simulink model "BLOC_ICE_control"  (R2016a)
settings: Solver=VariableStepAuto  StartTime=0.0  StopTime=10.0  RelTol=1e-3
undefined symbols (not defined in the file): DiscIntNeverNeededParam, fa_delta_derating, fa_high_derating_point, fa_kp_idle_tr_off, fa_kp_idle_tr_on, fa_low_derating_point, fa_max_tq_ice, fa_n_ice, fa_taui_idle_tr_off, fa_taui_idle_tr_on, fa_tq_loss, fa_tq_max_speed, hev_dt
libraries: simulink x3
settings Model: Creator=Florent  LastModifiedBy=Florent
settings OptimizationCC: DefaultParameterBehavior=Inlined  OptimizeModelRefInitCode=on  LifeSpan=1
settings RTWCC: SystemTargetFile=ert.tlc  TemplateMakefile=ert_default_tmf  GenerateReport=on  IncludeHyperlinkInReport=on  LaunchReport=on  TargetLang=C++  GenerateTraceInfo=on  GenerateTraceReport=on  GenerateTraceReportSl=on  GenerateTraceReportSf=on  GenerateTraceReportEml=on
settings CodeAppCC: ForceParamTrailComments=on  OperatorAnnotations=on  SimulinkDataObjDesc=on  SFDataObjDesc=on  MATLABFcnDesc=on  InsertBlockDesc=on  MATLABSourceComments=on
settings ERTTargetCC: GenerateSampleERTMain=on  MultiInstanceERTCode=on  CodeInterfacePackaging=C++ class  InlinedParameterPlacement=NonHierarchical  RootIOFormat=Structure reference  ERTCustomFileTemplate=example_file_process.tlc

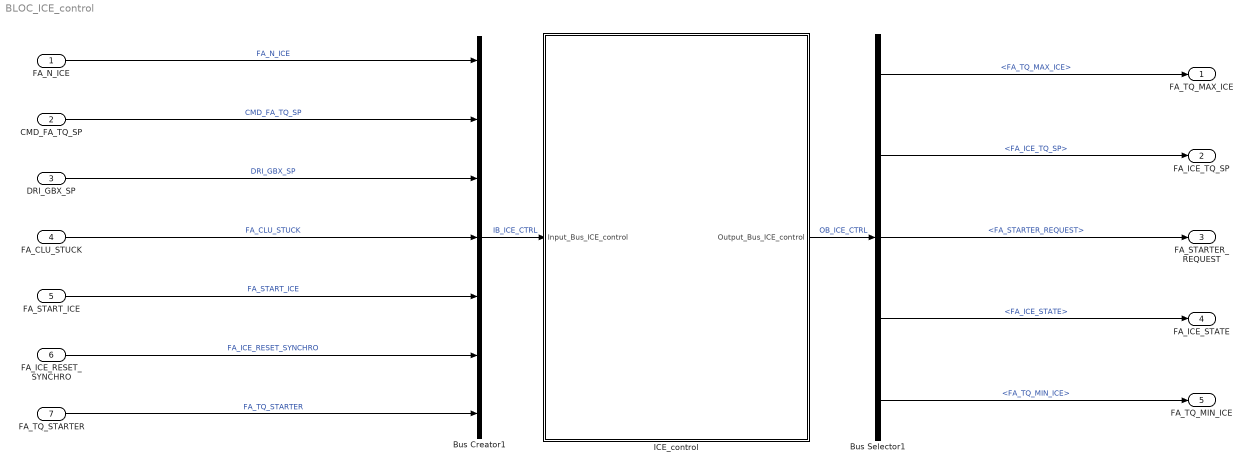
== system BLOC_ICE_control ==
  FA_N_ICE : Inport
  CMD_FA_TQ_SP : Inport  Port=2
  DRI_GBX_SP : Inport  Port=3
  FA_CLU_STUCK : Inport  Port=4
  FA_START_ICE : Inport  Port=5
  FA_ICE_RESET_SYNCHRO : Inport  Port=6
  FA_TQ_STARTER : Inport  Port=7
  Bus Creator1 : BusCreator  Inputs=7
  Bus Selector1 : BusSelector  OutputSignals=FA_TQ_MAX_ICE,FA_ICE_TQ_SP,FA_STARTER_REQUEST,FA_ICE_STATE,FA_TQ_MIN_ICE
  ICE_control : Subsystem  TreatAsAtomicUnit=on  SystemSampleTime=hev_dt
  FA_TQ_MAX_ICE : Outport
  FA_ICE_TQ_SP : Outport  Port=2
  FA_STARTER_REQUEST : Outport  Port=3
  FA_ICE_STATE : Outport  Port=4
  FA_TQ_MIN_ICE : Outport  Port=5
  wires:
  FA_N_ICE/1 -> Bus Creator1/1  "FA_N_ICE"
  CMD_FA_TQ_SP/1 -> Bus Creator1/2  "CMD_FA_TQ_SP"
  DRI_GBX_SP/1 -> Bus Creator1/3  "DRI_GBX_SP"
  FA_CLU_STUCK/1 -> Bus Creator1/4  "FA_CLU_STUCK"
  FA_START_ICE/1 -> Bus Creator1/5  "FA_START_ICE"
  FA_ICE_RESET_SYNCHRO/1 -> Bus Creator1/6  "FA_ICE_RESET_SYNCHRO"
  Bus Creator1/1 -> ICE_control/1("Input_Bus_ICE_control ")  "IB_ICE_CTRL"
  ICE_control/1(Output_Bus_ICE_control) -> Bus Selector1/1  "OB_ICE_CTRL"
  Bus Selector1/1 -> FA_TQ_MAX_ICE/1  "<FA_TQ_MAX_ICE>"
  Bus Selector1/2 -> FA_ICE_TQ_SP/1  "<FA_ICE_TQ_SP>"
  Bus Selector1/3 -> FA_STARTER_REQUEST/1  "<FA_STARTER_REQUEST>"
  Bus Selector1/4 -> FA_ICE_STATE/1  "<FA_ICE_STATE>"
  Bus Selector1/5 -> FA_TQ_MIN_ICE/1  "<FA_TQ_MIN_ICE>"
  FA_TQ_STARTER/1 -> Bus Creator1/7  "FA_TQ_STARTER"

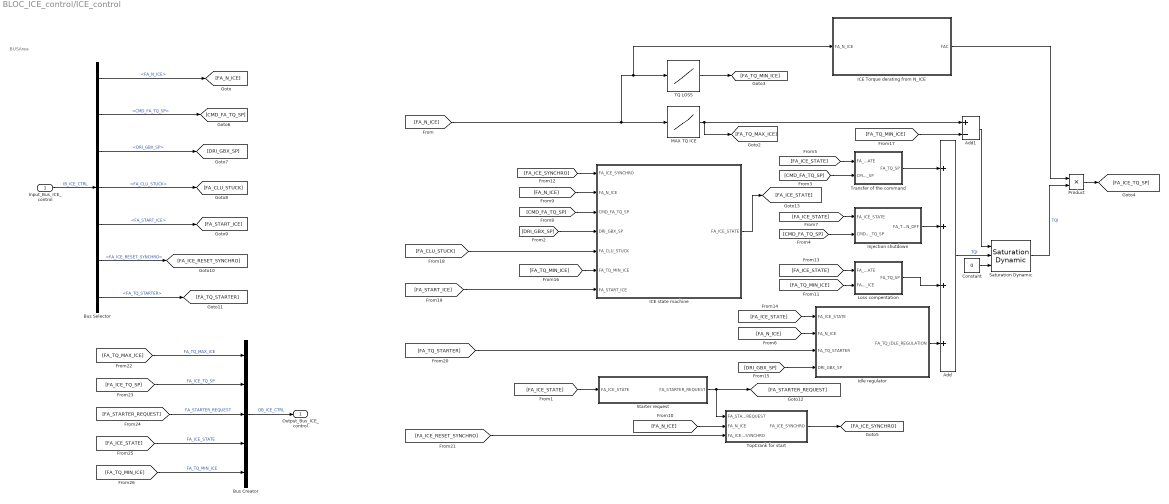
== system BLOC_ICE_control/ICE_control ==
  note: BUSArea
  "Input_Bus_ICE_control " : Inport
  Add : Sum  Inputs=4  SampleTime=hev_dt
  Add1 : Sum  Inputs=+-  SampleTime=hev_dt
  Bus Creator : BusCreator  Inputs=5
  Bus Selector : BusSelector  OutputSignals=FA_N_ICE,CMD_FA_TQ_SP,DRI_GBX_SP,FA_CLU_STUCK,FA_START_ICE,FA_ICE_RESET_SYNCHRO,FA_TQ_STARTER
  Constant : Constant  Value=0
  ICE Torque derating from N_ICE : Subsystem
  ICE state machine : Stateflow chart  TreatAsAtomicUnit=on
  Idle regulator : Subsystem
  Injection shutdown : Subsystem
  Loss compentation : Subsystem
  MAX TQ ICE : Lookup_n-D  NumberOfTableDimensions=1  BreakpointsForDimension1=fa_tq_max_speed  Table=fa_max_tq_ice  ExtrapMethod=Clip  UseLastTableValue=on  SampleTime=hev_dt  RndMeth=Simplest  InputSameDT=on
  Product : Product
  Saturation Dynamic : simulink/Discontinuities/Saturation Dynamic  OutMin=[]  OutMax=[]  OutDataTypeStr=Inherit: Same as second input  OutDataType=fixdt(1, 16)  OutScaling=2^-10  DoSatur=off
  Starter request : Subsystem
  TQ LOSS : Lookup_n-D  NumberOfTableDimensions=1  BreakpointsForDimension1=fa_n_ice  Table=fa_tq_loss  UseLastTableValue=on  SampleTime=hev_dt  RndMeth=Simplest  InputSameDT=on
  TopCrank for start : Subsystem
  Transfer of the command : Subsystem
  Output_Bus_ICE_control : Outport
  wires:
  [DRI_GBX_SP] -> ICE state machine/4(DRI_GBX_SP)
  ICE state machine/1(FA_ICE_STATE) -> [FA_ICE_STATE]
  Injection shutdown/1(FA_TQ_SP_INJECTION_OFF) -> Add/2
  Transfer of the command/1(FA_TQ_SP) -> Add/1
  [FA_ICE_STATE] -> Transfer of the command/1(FA_ICE_STATE)
  [CMD_FA_TQ_SP] -> Injection shutdown/2(CMD_FA_TQ_SP)
  Starter request/1(FA_STARTER_REQUEST) -> [FA_STARTER_REQUEST], TopCrank for start/1(FA_STARTER_REQUEST)
  [FA_ICE_STATE] -> Starter request/1(FA_ICE_STATE)
  Add/1 -> Saturation Dynamic/2  "TQI"
  MAX TQ ICE/1 -> [FA_TQ_MAX_ICE], Add1/1
  [CMD_FA_TQ_SP] -> ICE state machine/3(CMD_FA_TQ_SP)
  [FA_N_ICE] -> MAX TQ ICE/1, ICE Torque derating from N_ICE/1(FA_N_ICE), TQ LOSS/1
  [FA_ICE_STATE] -> Injection shutdown/1(FA_ICE_STATE)
  [FA_CLU_STUCK] -> ICE state machine/5(FA_CLU_STUCK)
  [FA_ICE_SYNCHRO] -> ICE state machine/1(FA_ICE_SYNCHRO)
  [FA_ICE_STATE] -> Loss compentation/1(FA_ICE_STATE)
  TopCrank for start/1(FA_ICE_SYNCHRO) -> [FA_ICE_SYNCHRO]
  Constant/1 -> Saturation Dynamic/3
  Add1/1 -> Saturation Dynamic/1
  [FA_ICE_RESET_SYNCHRO] -> TopCrank for start/3(FA_ICE_RESET_SYNCHRO)
  [FA_START_ICE] -> ICE state machine/7(FA_START_ICE)
  Saturation Dynamic/1 -> Product/2  "TQI"
  Loss compentation/1(FA_TQ_SP) -> Add/3
  [FA_ICE_STATE] -> Idle regulator/1(FA_ICE_STATE)
  [DRI_GBX_SP] -> Idle regulator/4(DRI_GBX_SP)
  Idle regulator/1(FA_TQ_IDLE_REGULATION) -> Add/4
  [FA_TQ_STARTER] -> Idle regulator/3(FA_TQ_STARTER)
  [FA_N_ICE] -> Idle regulator/2(FA_N_ICE)
  [FA_N_ICE] -> ICE state machine/2(FA_N_ICE)
  TQ LOSS/1 -> [FA_TQ_MIN_ICE]
  [FA_N_ICE] -> TopCrank for start/2(FA_N_ICE)
  [FA_TQ_MIN_ICE] -> Loss compentation/2(FA_TQ_MIN_ICE)
  [FA_TQ_MIN_ICE] -> ICE state machine/6(FA_TQ_MIN_ICE)
  [FA_TQ_MIN_ICE] -> Add1/2
  [CMD_FA_TQ_SP] -> Transfer of the command/2(CMD_FA_TQ_SP)
  ICE Torque derating from N_ICE/1(FAC) -> Product/1
  Product/1 -> [FA_ICE_TQ_SP]
  "Input_Bus_ICE_control "/1 -> Bus Selector/1  "IB_ICE_CTRL"
  Bus Selector/1 -> [FA_N_ICE]  "<FA_N_ICE>"
  Bus Selector/2 -> [CMD_FA_TQ_SP]  "<CMD_FA_TQ_SP>"
  Bus Selector/3 -> [DRI_GBX_SP]  "<DRI_GBX_SP>"
  Bus Selector/4 -> [FA_CLU_STUCK]  "<FA_CLU_STUCK>"
  Bus Selector/5 -> [FA_START_ICE]  "<FA_START_ICE>"
  Bus Selector/6 -> [FA_ICE_RESET_SYNCHRO]  "<FA_ICE_RESET_SYNCHRO>"
  Bus Selector/7 -> [FA_TQ_STARTER]  "<FA_TQ_STARTER>"
  Bus Creator/1 -> Output_Bus_ICE_control/1  "OB_ICE_CTRL"
  [FA_TQ_MAX_ICE] -> Bus Creator/1  "FA_TQ_MAX_ICE"
  [FA_ICE_TQ_SP] -> Bus Creator/2  "FA_ICE_TQ_SP"
  [FA_STARTER_REQUEST] -> Bus Creator/3  "FA_STARTER_REQUEST"
  [FA_ICE_STATE] -> Bus Creator/4  "FA_ICE_STATE"
  [FA_TQ_MIN_ICE] -> Bus Creator/5  "FA_TQ_MIN_ICE"

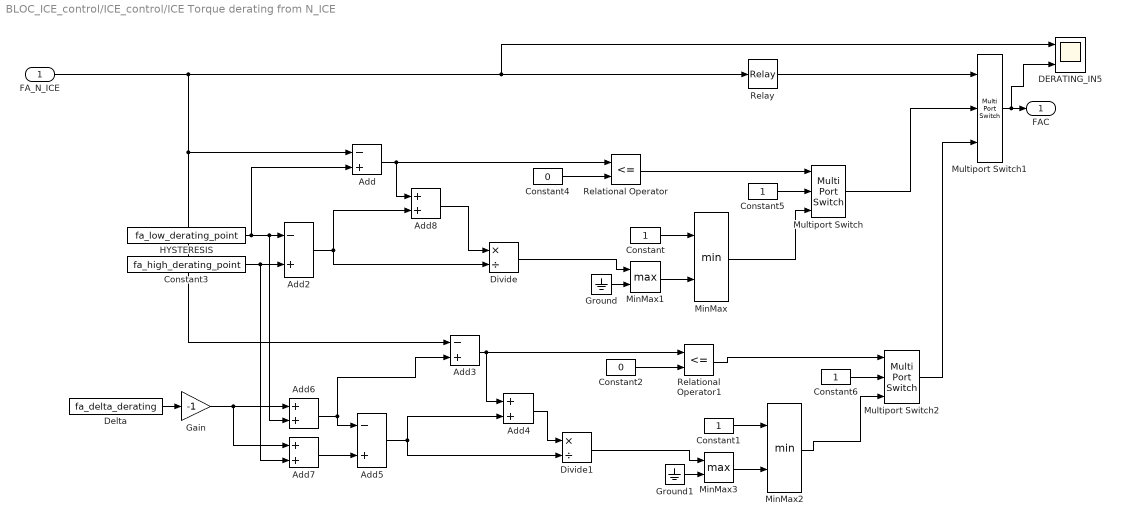
== system BLOC_ICE_control/ICE_control/ICE Torque derating from N_ICE ==
  FA_N_ICE : Inport
  Add{,2..3,5} (4 alike) : Sum  Inputs=-+
  Add{4,6..8} (4 alike) : Sum
  Constant{,1,5..6} (4 alike) : Constant
  Constant2 : Constant  Value=0
  Constant3 : Constant  Value=fa_high_derating_point
  Constant4 : Constant  Value=0
  DERATING_IN5 : Scope  NumInputPorts=2
  Delta : Constant  Value=fa_delta_derating
  Divide : Product  Inputs=*/
  Divide1 : Product  Inputs=*/
  Gain : Gain  Gain=-1
  Ground : Ground
  Ground1 : Ground
  HYSTERESIS : Constant  Value=fa_low_derating_point
  MinMax : MinMax  Inputs=2
  MinMax1 : MinMax  Function=max  Inputs=2
  MinMax2 : MinMax  Inputs=2
  MinMax3 : MinMax  Function=max  Inputs=2
  Multiport Switch : MultiPortSwitch  DataPortOrder=Zero-based contiguous  Inputs=2
  Multiport Switch1 : MultiPortSwitch  DataPortOrder=Zero-based contiguous  Inputs=2
  Multiport Switch2 : MultiPortSwitch  DataPortOrder=Zero-based contiguous  Inputs=2
  Relational Operator : RelationalOperator  Operator=<=  OutDataTypeStr=boolean
  Relational Operator1 : RelationalOperator  Operator=<=  OutDataTypeStr=boolean
  Relay : Relay  OnSwitchValue=5750  OffSwitchValue=4900-500
  FAC : Outport
  wires:
  Gain/1 -> Add6/1, Add7/1
  Add4/1 -> Divide1/1
  Add8/1 -> Divide/1
  Add7/1 -> Add5/2
  Add6/1 -> Add3/2, Add5/1
  Constant6/1 -> Multiport Switch2/2
  MinMax2/1 -> Multiport Switch2/3
  Relational Operator1/1 -> Multiport Switch2/1
  Constant2/1 -> Relational Operator1/2
  Add3/1 -> Relational Operator1/1, Add4/1
  Divide1/1 -> MinMax3/1
  MinMax3/1 -> MinMax2/2
  Ground1/1 -> MinMax3/2
  Constant1/1 -> MinMax2/1
  FA_N_ICE/1 -> Add3/1, Add/1, Relay/1, DERATING_IN5/1
  Delta/1 -> Gain/1
  Constant3/1 -> Add2/2, Add7/2
  Multiport Switch2/1 -> Multiport Switch1/3
  HYSTERESIS/1 -> Add6/2, Add2/1, Add/2
  Multiport Switch/1 -> Multiport Switch1/2
  Constant5/1 -> Multiport Switch/2
  MinMax/1 -> Multiport Switch/3
  Relational Operator/1 -> Multiport Switch/1
  Constant4/1 -> Relational Operator/2
  Add/1 -> Add8/1, Relational Operator/1
  Relay/1 -> Multiport Switch1/1
  Divide/1 -> MinMax1/1
  MinMax1/1 -> MinMax/2
  Ground/1 -> MinMax1/2
  Constant/1 -> MinMax/1
  Multiport Switch1/1 -> FAC/1, DERATING_IN5/2
  Add2/1 -> Divide/2, Add8/2
  Add5/1 -> Divide1/2, Add4/2

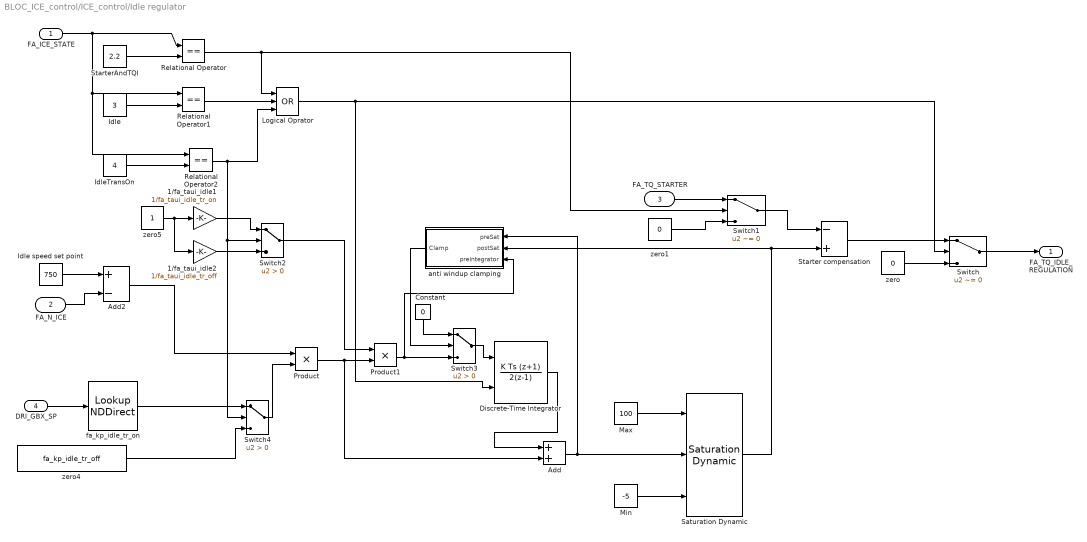
== system BLOC_ICE_control/ICE_control/Idle regulator ==
  FA_ICE_STATE : Inport
  FA_N_ICE : Inport  Port=2
  FA_TQ_STARTER : Inport  Port=3
  DRI_GBX_SP : Inport  Port=4
  1/fa_taui_idle1 : Gain  Gain=1/fa_taui_idle_tr_on  SampleTime=hev_dt
  1/fa_taui_idle2 : Gain  Gain=1/fa_taui_idle_tr_off  SampleTime=hev_dt
  Add : Sum  SampleTime=hev_dt
  Add2 : Sum  Inputs=+-  SampleTime=hev_dt
  Constant : Constant  DisableCoverage=on  Value=0  OutDataTypeStr=Inherit: Inherit via back propagation  PreserveConstantTs=on
  Discrete-Time Integrator : DiscreteIntegrator  IntegratorMethod=Integration: Trapezoidal  ExternalReset=rising  SampleTime=hev_dt  ICPrevOutput=DiscIntNeverNeededParam  ICPrevScaledInput=DiscIntNeverNeededParam
  Idle : Constant  Value=3
  Idle speed set point : Constant  Value=750
  IdleTransOn : Constant  Value=4
  Logical Oprator : Logic  Operator=OR  Inputs=3  AllPortsSameDT=off  OutDataTypeStr=boolean  SampleTime=hev_dt
  Max : Constant  Value=100
  Min : Constant  Value=-5
  Product : Product  SampleTime=hev_dt  RndMeth=Zero
  Product1 : Product  SampleTime=hev_dt  RndMeth=Zero
  Relational Operator : RelationalOperator  Operator===  OutDataTypeStr=boolean  SampleTime=hev_dt
  Relational Operator1 : RelationalOperator  Operator===  OutDataTypeStr=boolean  SampleTime=hev_dt
  Relational Operator2 : RelationalOperator  Operator===  OutDataTypeStr=boolean  SampleTime=hev_dt
  Saturation Dynamic : simulink/Discontinuities/Saturation Dynamic  OutMin=[]  OutMax=[]  OutDataTypeStr=Inherit: Same as second input  OutDataType=fixdt(1, 16)  OutScaling=2^-10  DoSatur=off
  Starter compensation : Sum  Inputs=-+  SampleTime=hev_dt
  StarterAndTQI : Constant  Value=2.2
  Switch : Switch  Criteria=u2 ~= 0  SampleTime=hev_dt
  Switch1 : Switch  Criteria=u2 ~= 0  SampleTime=hev_dt
  Switch2 : Switch  DisableCoverage=on  Criteria=u2 > Threshold  SampleTime=hev_dt  InputSameDT=on
  Switch3 : Switch  DisableCoverage=on  Criteria=u2 > Threshold  SampleTime=hev_dt  InputSameDT=on
  Switch4 : Switch  DisableCoverage=on  Criteria=u2 > Threshold  SampleTime=hev_dt  InputSameDT=on
  anti windup clamping : Subsystem
  fa_kp_idle_tr_on : LookupNDDirect  NumberOfTableDimensions=1  Table=fa_kp_idle_tr_on  SampleTime=hev_dt
  zero : Constant  Value=0
  zero1 : Constant  Value=0
  zero4 : Constant  Value=fa_kp_idle_tr_off
  zero5 : Constant
  FA_TQ_IDLE_REGULATION : Outport
  wires:
  FA_ICE_STATE/1 -> Relational Operator/1, Relational Operator1/1, Relational Operator2/1
  Switch/1 -> FA_TQ_IDLE_REGULATION/1
  zero/1 -> Switch/3
  Idle speed set point/1 -> Add2/1
  FA_N_ICE/1 -> Add2/2
  Relational Operator1/1 -> Logical Oprator/2
  StarterAndTQI/1 -> Relational Operator/2
  Idle/1 -> Relational Operator1/2
  zero1/1 -> Switch1/3
  FA_TQ_STARTER/1 -> Switch1/1
  IdleTransOn/1 -> Relational Operator2/2
  Starter compensation/1 -> Switch/1
  Logical Oprator/1 -> Switch/2, Discrete-Time Integrator/2
  anti windup clamping/1(Clamp) -> Switch3/2
  Constant/1 -> Switch3/1
  Product1/1 -> anti windup clamping/3(preIntegrator), Switch3/3
  zero5/1 -> 1/fa_taui_idle1/1, 1/fa_taui_idle2/1
  1/fa_taui_idle1/1 -> Switch2/1
  1/fa_taui_idle2/1 -> Switch2/3
  DRI_GBX_SP/1 -> fa_kp_idle_tr_on/1
  Product/1 -> Add/2, Product1/2
  Add2/1 -> Product/1
  fa_kp_idle_tr_on/1 -> Switch4/1
  Switch2/1 -> Product1/1
  zero4/1 -> Switch4/3
  Switch4/1 -> Product/2
  Relational Operator2/1 -> Logical Oprator/3, Switch4/2, Switch2/2
  Switch1/1 -> Starter compensation/1
  Discrete-Time Integrator/1 -> Add/1
  Relational Operator/1 -> Switch1/2, Logical Oprator/1
  Switch3/1 -> Discrete-Time Integrator/1
  Min/1 -> Saturation Dynamic/3
  Max/1 -> Saturation Dynamic/1
  Add/1 -> Saturation Dynamic/2, anti windup clamping/1(preSat)
  Saturation Dynamic/1 -> Starter compensation/2, anti windup clamping/2(postSat)

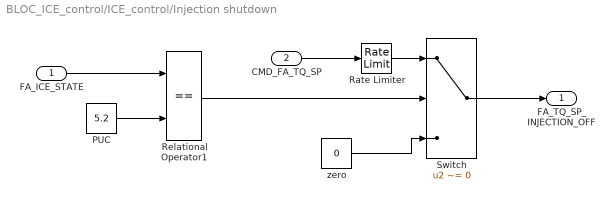
== system BLOC_ICE_control/ICE_control/Injection shutdown ==
  FA_ICE_STATE : Inport
  CMD_FA_TQ_SP : Inport  Port=2
  PUC : Constant  Value=5.2
  Rate Limiter : RateLimiter  RisingSlewLimit=20  FallingSlewLimit=-100  SampleTimeMode=inherited
  Relational Operator1 : RelationalOperator  Operator===  OutDataTypeStr=boolean  SampleTime=hev_dt
  Switch : Switch  Criteria=u2 ~= 0  SampleTime=hev_dt
  zero : Constant  Value=0
  FA_TQ_SP_INJECTION_OFF : Outport
  wires:
  Relational Operator1/1 -> Switch/2
  Rate Limiter/1 -> Switch/1
  FA_ICE_STATE/1 -> Relational Operator1/1
  CMD_FA_TQ_SP/1 -> Rate Limiter/1
  PUC/1 -> Relational Operator1/2
  Switch/1 -> FA_TQ_SP_INJECTION_OFF/1
  zero/1 -> Switch/3

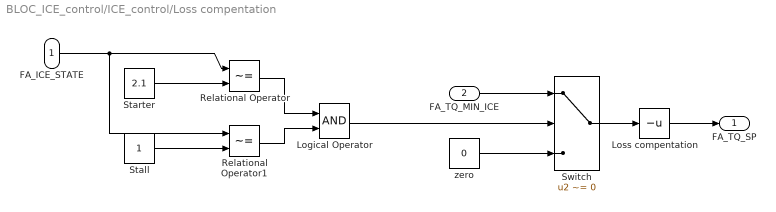
== system BLOC_ICE_control/ICE_control/Loss compentation ==
  FA_ICE_STATE : Inport
  FA_TQ_MIN_ICE : Inport  Port=2
  Logical Operator : Logic  AllPortsSameDT=off  OutDataTypeStr=boolean  SampleTime=hev_dt
  Loss compentation : UnaryMinus  SampleTime=hev_dt
  Relational Operator : RelationalOperator  Operator=~=  OutDataTypeStr=boolean  SampleTime=hev_dt
  Relational Operator1 : RelationalOperator  Operator=~=  OutDataTypeStr=boolean  SampleTime=hev_dt
  Stall : Constant
  Starter : Constant  Value=2.1
  Switch : Switch  Criteria=u2 ~= 0  SampleTime=hev_dt
  zero : Constant  Value=0
  FA_TQ_SP : Outport
  wires:
  FA_TQ_MIN_ICE/1 -> Switch/1
  zero/1 -> Switch/3
  Switch/1 -> Loss compentation/1
  Stall/1 -> Relational Operator1/2
  Starter/1 -> Relational Operator/2
  FA_ICE_STATE/1 -> Relational Operator/1, Relational Operator1/1
  Relational Operator/1 -> Logical Operator/1
  Relational Operator1/1 -> Logical Operator/2
  Loss compentation/1 -> FA_TQ_SP/1
  Logical Operator/1 -> Switch/2

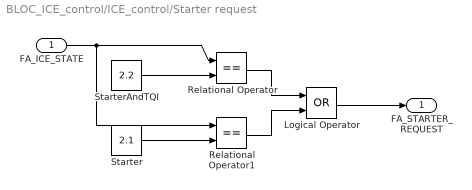
== system BLOC_ICE_control/ICE_control/Starter request ==
  FA_ICE_STATE : Inport
  Logical Operator : Logic  Operator=OR  AllPortsSameDT=off  OutDataTypeStr=boolean  SampleTime=hev_dt
  Relational Operator : RelationalOperator  Operator===  OutDataTypeStr=boolean  SampleTime=hev_dt
  Relational Operator1 : RelationalOperator  Operator===  OutDataTypeStr=boolean  SampleTime=hev_dt
  Starter : Constant  Value=2.1
  StarterAndTQI : Constant  Value=2.2
  FA_STARTER_REQUEST : Outport
  wires:
  Relational Operator1/1 -> Logical Operator/2
  Relational Operator/1 -> Logical Operator/1
  FA_ICE_STATE/1 -> Relational Operator1/1, Relational Operator/1
  StarterAndTQI/1 -> Relational Operator/2
  Starter/1 -> Relational Operator1/2
  Logical Operator/1 -> FA_STARTER_REQUEST/1

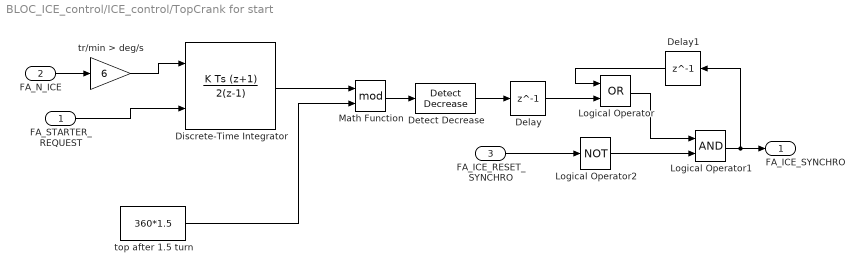
== system BLOC_ICE_control/ICE_control/TopCrank for start ==
  FA_STARTER_REQUEST : Inport
  FA_N_ICE : Inport  Port=2
  FA_ICE_RESET_SYNCHRO : Inport  Port=3
  Delay : Delay  DelayLength=1  SampleTime=hev_dt
  Delay1 : Delay  DelayLength=1  SampleTime=hev_dt
  Detect Decrease : simulink/Logic and Bit Operations/Detect Decrease  vinit=0.0  InputProcessing=Inherited  OutDataTypeStr=uint8
  Discrete-Time Integrator : DiscreteIntegrator  IntegratorMethod=Integration: Trapezoidal  ExternalReset=rising  SampleTime=hev_dt  ICPrevOutput=DiscIntNeverNeededParam  ICPrevScaledInput=DiscIntNeverNeededParam
  Logical Operator : Logic  Operator=OR  AllPortsSameDT=off  OutDataTypeStr=boolean  SampleTime=hev_dt
  Logical Operator1 : Logic  AllPortsSameDT=off  OutDataTypeStr=boolean  SampleTime=hev_dt
  Logical Operator2 : Logic  Operator=NOT  AllPortsSameDT=off  OutDataTypeStr=boolean  SampleTime=hev_dt
  Math Function : Math  Operator=mod  SampleTime=hev_dt  SaturateOnIntegerOverflow=on
  top after 1.5 turn : Constant  Value=360*1.5
  tr/min > deg/s : Gain  Gain=6  SampleTime=hev_dt
  FA_ICE_SYNCHRO : Outport
  wires:
  tr/min > deg/s/1 -> Discrete-Time Integrator/1
  Discrete-Time Integrator/1 -> Math Function/1
  top after 1.5 turn/1 -> Math Function/2
  Math Function/1 -> Detect Decrease/1
  Detect Decrease/1 -> Delay/1
  FA_N_ICE/1 -> tr/min > deg/s/1
  FA_STARTER_REQUEST/1 -> Discrete-Time Integrator/2
  Logical Operator/1 -> Logical Operator1/1
  FA_ICE_RESET_SYNCHRO/1 -> Logical Operator2/1
  Logical Operator2/1 -> Logical Operator1/2
  Delay1/1 -> Logical Operator/1
  Logical Operator1/1 -> Delay1/1, FA_ICE_SYNCHRO/1
  Delay/1 -> Logical Operator/2

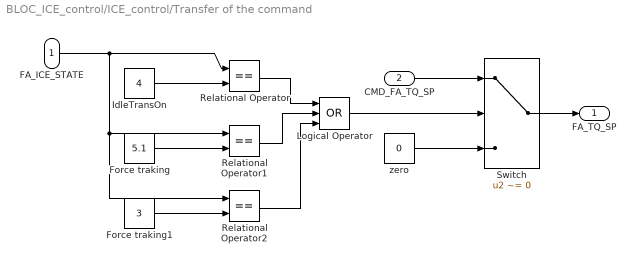
== system BLOC_ICE_control/ICE_control/Transfer of the command ==
  FA_ICE_STATE : Inport
  CMD_FA_TQ_SP : Inport  Port=2
  Force traking : Constant  Value=5.1  VectorParams1D=off
  Force traking1 : Constant  Value=3  VectorParams1D=off
  IdleTransOn : Constant  Value=4
  Logical Operator : Logic  Operator=OR  Inputs=3  AllPortsSameDT=off  OutDataTypeStr=boolean  SampleTime=hev_dt
  Relational Operator : RelationalOperator  Operator===  OutDataTypeStr=boolean  SampleTime=hev_dt
  Relational Operator1 : RelationalOperator  Operator===  OutDataTypeStr=boolean  SampleTime=hev_dt
  Relational Operator2 : RelationalOperator  Operator===  OutDataTypeStr=boolean  SampleTime=hev_dt
  Switch : Switch  Criteria=u2 ~= 0  SampleTime=hev_dt
  zero : Constant  Value=0
  FA_TQ_SP : Outport
  wires:
  Relational Operator1/1 -> Logical Operator/2
  Relational Operator/1 -> Logical Operator/1
  FA_ICE_STATE/1 -> Relational Operator/1, Relational Operator1/1, Relational Operator2/1
  IdleTransOn/1 -> Relational Operator/2
  Force traking/1 -> Relational Operator1/2
  Logical Operator/1 -> Switch/2
  Switch/1 -> FA_TQ_SP/1
  zero/1 -> Switch/3
  CMD_FA_TQ_SP/1 -> Switch/1
  Force traking1/1 -> Relational Operator2/2
  Relational Operator2/1 -> Logical Operator/3

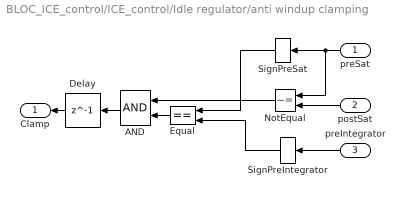
== system BLOC_ICE_control/ICE_control/Idle regulator/anti windup clamping ==
  preSat : Inport
  postSat : Inport  Port=2
  preIntegrator : Inport  Port=3
  AND : Logic  DisableCoverage=on  OutDataTypeStr=boolean  SampleTime=hev_dt
  Delay : Delay  DelayLength=1  SampleTime=hev_dt
  Equal : RelationalOperator  DisableCoverage=on  Operator===  OutDataTypeStr=boolean  SampleTime=hev_dt  InputSameDT=on
  NotEqual : RelationalOperator  DisableCoverage=on  Operator=~=  OutDataTypeStr=boolean  SampleTime=hev_dt  InputSameDT=on
  SignPreIntegrator : Signum  DisableCoverage=on  SampleTime=hev_dt
  SignPreSat : Signum  DisableCoverage=on  SampleTime=hev_dt
  Clamp : Outport
  wires:
  preSat/1 -> SignPreSat/1, NotEqual/1
  postSat/1 -> NotEqual/2
  preIntegrator/1 -> SignPreIntegrator/1
  SignPreSat/1 -> Equal/1
  NotEqual/1 -> AND/1
  SignPreIntegrator/1 -> Equal/2
  Equal/1 -> AND/2
  AND/1 -> Delay/1
  Delay/1 -> Clamp/1

== stateflow chart BLOC_ICE_control/ICE_control/ICE state machine ==
  state Start
    state Starter
      en: FA_ICE_STATE=2.1;
    state StarterAndTQI
      en: FA_ICE_STATE=2.2;
    (default) -> Starter
    Starter -> StarterAndTQI : [(FA_N_ICE>250)&&(FA_ICE_SYNCHRO==1)]
  state Stall
    en: FA_ICE_STATE=1;
  state Running
    state Idle
      en: FA_ICE_STATE=3;
    state IdleTransOn
      en: FA_ICE_STATE=4;
    state Force_tracking
      state Standard_force_tracking
        en: FA_ICE_STATE=5.1;
      state InjectionInhibed
        en: FA_ICE_STATE=5.2;
      (default) -> Standard_force_tracking
      InjectionInhibed -> Standard_force_tracking [order 1] : [CMD_FA_TQ_SP>FA_TQ_MIN_ICE]
      Standard_force_tracking -> InjectionInhibed : [(CMD_FA_TQ_SP==FA_TQ_MIN_ICE)]
    (default) -> (junction 111)
    (junction 111) -> IdleTransOn [order 1] : [(FA_CLU_STUCK!=0)&&(DRI_GBX_SP!=0)]
    (junction 111) -> Idle [order 2]
    IdleTransOn -> Idle [order 1] : [((FA_CLU_STUCK==0)||(DRI_GBX_SP==0))]
    Idle -> IdleTransOn : [(FA_CLU_STUCK!=0)&&(DRI_GBX_SP!=0)]
    Force_tracking -> Idle : [((FA_CLU_STUCK==0)||(DRI_GBX_SP==0))]
    IdleTransOn -> Force_tracking [order 2] : [(FA_CLU_STUCK==1)&&(DRI_GBX_SP!=0)&&(CMD_FA_TQ_SP>0)]
    InjectionInhibed -> IdleTransOn [order 2] : [(FA_N_ICE<1200)&&(FA_CLU_STUCK==1)&&(DRI_GBX_SP!=0)]
  (default) -> Stall
  Start -> Stall [order 2] : [FA_START_ICE!=1]
  Stall -> Start [order 1] : [(FA_START_ICE==1)&&(FA_N_ICE<30)]
  Stall -> Force_tracking [order 2] : [(FA_START_ICE==1)&&(FA_N_ICE>600)&&(DRI_GBX_SP!=0)&&(FA_CLU_STUCK==1)]
  Running -> Stall : [(FA_START_ICE!=1)||(FA_N_ICE<400)]
  StarterAndTQI -> Stall : [(FA_N_ICE<250)]
  Start -> Running [order 1] : [FA_N_ICE>600]
  data: FA_ICE_SYNCHRO input; FA_N_ICE input double; CMD_FA_TQ_SP input double; DRI_GBX_SP input double; FA_ICE_STATE output double; FA_CLU_STUCK input; FA_TQ_MIN_ICE input double; FA_START_ICE input double
